simulink model "Pid"  (R2018a)
settings: Solver=VariableStepAuto  StartTime=0.0  StopTime=inf  RelTol=1e-3
undefined symbols (not defined in the file or in its folder): f
libraries: simulink x26, instrumentlib x3, aerolibanimutils x1
settings Model: Creator=user  LastModifiedBy=user

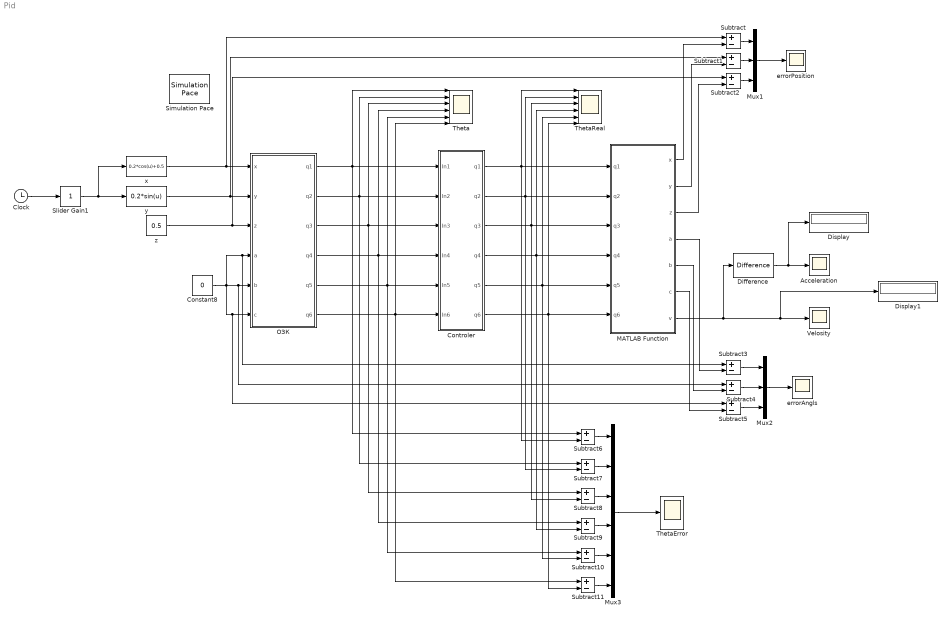
== system Pid ==
  Acceleration : Scope
  Clock : Clock
  Constant8 : Constant  Value=0
  Controler : Subsystem
  Difference : simulink/Discrete/Difference  ICPrevInput=0.0  OutMin=[]  OutMax=[]  OutDataType=fixdt(1, 16)  OutScaling=2^-10  DoSatur=off
  Display : Display
  Display1 : Display
  MATLAB Function : MATLAB Function  TreatAsAtomicUnit=on
  Mux1 : Mux  Inputs=3
  Mux2 : Mux  Inputs=3
  Mux3 : Mux  Inputs=6
  Simulation Pace : aerolibanimutils/Simulation Pace  SimulationPace=1  SleepMode=MATLAB Thread  OutputPaceError=off  SampleTime=1/200
  Slider Gain1 : simulink/Math Operations/Slider Gain  gain=1  low=0  high=10
  Subtract{,1..11} (12 alike) : Sum  Inputs=+-
  Theta : Scope  NumInputPorts=6
  ThetaError : Scope
  ThetaReal : Scope  NumInputPorts=6
  Velosity : Scope
  errorAngls : Scope
  errorPosition : Scope
  x : Fcn  Expr=0.2*cos(u)+0.5
  y : Fcn  Expr=0.2*sin(u)
  z : Constant  Value=0.5
  ОЗК : MATLAB Function  TreatAsAtomicUnit=on
  wires:
  Constant8/1 -> Subtract3/1, ОЗК/4(a), Subtract5/1, ОЗК/6(c), Subtract4/1, ОЗК/5(b)
  MATLAB Function/1(x) -> Subtract/2
  MATLAB Function/2(y) -> Subtract1/2
  MATLAB Function/3(z) -> Subtract2/2
  MATLAB Function/4(a) -> Subtract3/2
  MATLAB Function/5(b) -> Subtract4/2
  MATLAB Function/6(c) -> Subtract5/2
  ОЗК/1(q1) -> Subtract6/1, Controler/1(In1), Theta/1
  ОЗК/3(q3) -> Subtract8/1, Theta/3, Controler/3(In3)
  ОЗК/4(q4) -> Subtract9/1, Controler/4(In4), Theta/4
  ОЗК/2(q2) -> Subtract7/1, Controler/2(In2), Theta/2
  ОЗК/5(q5) -> Subtract10/1, Theta/5, Controler/5(In5)
  ОЗК/6(q6) -> Subtract11/1, Controler/6(In6), Theta/6
  z/1 -> Subtract2/1, ОЗК/3(z)
  y/1 -> Subtract1/1, ОЗК/2(y)
  x/1 -> Subtract/1, ОЗК/1(x)
  Controler/1("q1 ") -> Subtract6/2, ThetaReal/1, MATLAB Function/1(q1)
  Controler/2(q2) -> Subtract7/2, ThetaReal/2, MATLAB Function/2(q2)
  Controler/3(q3) -> Subtract8/2, ThetaReal/3, MATLAB Function/3(q3)
  Controler/4(q4) -> Subtract9/2, ThetaReal/4, MATLAB Function/4(q4)
  Controler/5(q5) -> Subtract10/2, ThetaReal/5, MATLAB Function/5(q5)
  Controler/6(q6) -> Subtract11/2, ThetaReal/6, MATLAB Function/6(q6)
  MATLAB Function/7(v) -> Difference/1, Display1/1, Velosity/1
  Difference/1 -> Display/1, Acceleration/1
  Subtract/1 -> Mux1/1
  Subtract1/1 -> Mux1/2
  Subtract2/1 -> Mux1/3
  Mux1/1 -> errorPosition/1
  Subtract4/1 -> Mux2/2
  Subtract3/1 -> Mux2/1
  Subtract5/1 -> Mux2/3
  Mux2/1 -> errorAngls/1
  Subtract6/1 -> Mux3/1
  Subtract7/1 -> Mux3/2
  Subtract8/1 -> Mux3/3
  Subtract9/1 -> Mux3/4
  Subtract10/1 -> Mux3/5
  Subtract11/1 -> Mux3/6
  Mux3/1 -> ThetaError/1
  Clock/1 -> Slider Gain1/1
  Slider Gain1/1 -> x/1, y/1

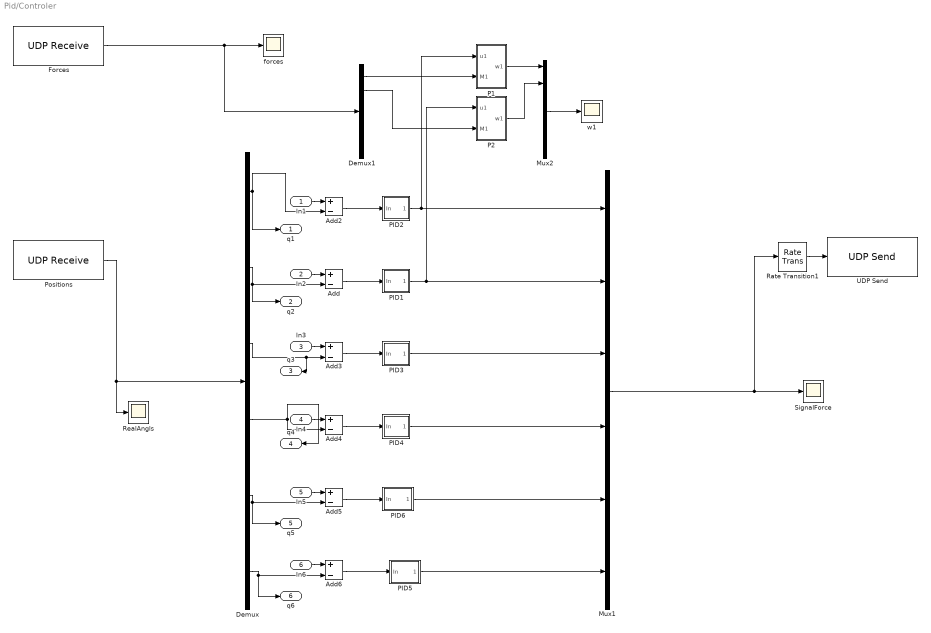
== system Pid/Controler ==
  In1 : Inport
  In2 : Inport  Port=2
  In3 : Inport  Port=3
  In4 : Inport  Port=4
  In5 : Inport  Port=5
  In6 : Inport  Port=6
  Add{,2..6} (6 alike) : Sum  Inputs=+-
  Demux : Demux  Outputs=6
  Demux1 : Demux  Outputs=6
  Forces : instrumentlib/UDP Receive  Host=localhost  Port=20005  LocalPort=20005  EnablePortSharing=off  GetLatestData=off  DataSize=6  DataType=double  ASCIIFormatting=%f,  Terminator=LF  ByteOrder=LittleEndian  EnableBlockingMode=on  Timeout=10  SampleTime=0.01  LocalAddress=localhost
      settings: SourceProductName=Instrument Control Toolbox
  Mux1 : Mux  Inputs=6
  Mux2 : Mux  Inputs=6
  P1 : Subsystem
  P2 : Subsystem
  PID1 : Subsystem
  PID2 : Subsystem
  PID3 : Subsystem
  PID4 : Subsystem
  PID5 : Subsystem
  PID6 : Subsystem
  Positions : instrumentlib/UDP Receive  Host=localhost  Port=20001  LocalPort=20001  EnablePortSharing=off  GetLatestData=off  DataSize=6  DataType=double  ASCIIFormatting=%f,  Terminator=LF  ByteOrder=LittleEndian  EnableBlockingMode=on  Timeout=10  SampleTime=0.01  LocalAddress=localhost
      settings: SourceProductName=Instrument Control Toolbox
  Rate Transition1 : RateTransition  OutPortSampleTime=0.01
  RealAngls : Scope
  SignalForce : Scope
  UDP Send : instrumentlib/UDP Send  Host=localhost  Port=20000  LocalPort=-1  EnablePortSharing=off  ByteOrder=LittleEndian  OutputDatagramPacketSize=512  EnableBlockingMode=on  LocalAddress=0.0.0.0
      settings: SourceProductName=Instrument Control Toolbox
  forces : Scope
  w1 : Scope
  "q1 " : Outport
  q2 : Outport  Port=2
  q3 : Outport  Port=3
  q4 : Outport  Port=4
  q5 : Outport  Port=5
  q6 : Outport  Port=6
  wires:
  Mux1/1 -> Rate Transition1/1, SignalForce/1
  In4/1 -> Add4/1
  In5/1 -> Add5/1
  Rate Transition1/1 -> UDP Send/1
  In3/1 -> Add3/1
  In1/1 -> Add2/1
  In6/1 -> Add6/1
  In2/1 -> Add/1
  PID2/1("out1 ") -> P1/1(u1), Mux1/1
  PID1/1("out1 ") -> P2/1(u1), Mux1/2
  PID3/1("out1 ") -> Mux1/3
  PID4/1("out1 ") -> Mux1/4
  PID6/1("out1 ") -> Mux1/5
  PID5/1("out1 ") -> Mux1/6
  Add/1 -> PID1/1(In)
  Add2/1 -> PID2/1(In)
  Add3/1 -> PID3/1(In)
  Add4/1 -> PID4/1(In)
  Add5/1 -> PID6/1(In)
  Add6/1 -> PID5/1(In)
  P1/1(w1) -> Mux2/1
  Mux2/1 -> w1/1
  Demux1/2 -> P2/2(M1)
  P2/1(w1) -> Mux2/2
  Positions/1 -> Demux/1, RealAngls/1
  Forces/1 -> Demux1/1, forces/1
  Demux/1 -> Add2/2, "q1 "/1
  Demux/2 -> Add/2, q2/1
  Demux/3 -> Add3/2, q3/1
  Demux/4 -> q4/1, Add4/2
  Demux/5 -> Add5/2, q5/1
  Demux/6 -> Add6/2, q6/1
  Demux1/1 -> P1/2(M1)

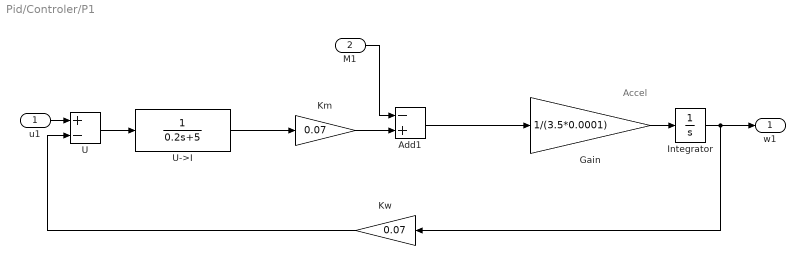
== system Pid/Controler/P1 ==
  note: Accel
  u1 : Inport
  M1 : Inport  Port=2
  Add1 : Sum  Inputs=-+
  Gain : Gain  Gain=1/(3.5*0.0001)
  Integrator : Integrator
  Km : Gain  Gain=0.07
  Kw : Gain  Gain=0.07
  U : Sum  Inputs=+-
  U->I : TransferFcn  Denominator=[0.2 5]
  w1 : Outport
  wires:
  U->I/1 -> Km/1
  Km/1 -> Add1/2
  u1/1 -> U/1
  Integrator/1 -> w1/1, Kw/1
  Kw/1 -> U/2
  U/1 -> U->I/1
  Gain/1 -> Integrator/1
  Add1/1 -> Gain/1
  M1/1 -> Add1/1

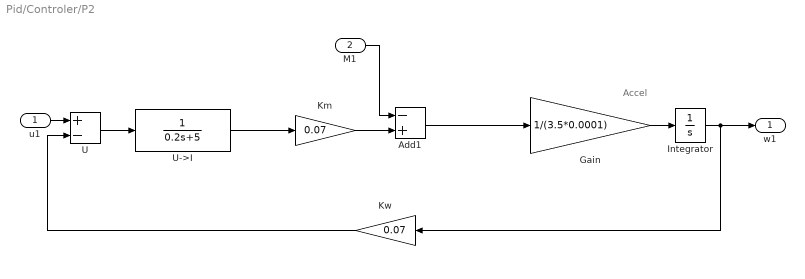
== system Pid/Controler/P2 ==
  note: Accel
  u1 : Inport
  M1 : Inport  Port=2
  Add1 : Sum  Inputs=-+
  Gain : Gain  Gain=1/(3.5*0.0001)
  Integrator : Integrator
  Km : Gain  Gain=0.07
  Kw : Gain  Gain=0.07
  U : Sum  Inputs=+-
  U->I : TransferFcn  Denominator=[0.2 5]
  w1 : Outport
  wires:
  M1/1 -> Add1/1
  Add1/1 -> Gain/1
  Gain/1 -> Integrator/1
  U/1 -> U->I/1
  Kw/1 -> U/2
  Integrator/1 -> Kw/1, w1/1
  u1/1 -> U/1
  Km/1 -> Add1/2
  U->I/1 -> Km/1

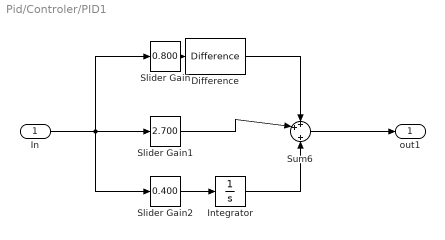
== system Pid/Controler/PID1 ==
  In : Inport
  Difference : simulink/Discrete/Difference  ICPrevInput=0.0  OutMin=[]  OutMax=[]  OutDataType=fixdt(1, 16)  OutScaling=2^-10  DoSatur=off
  Integrator : Integrator
  Slider Gain : simulink/Math Operations/Slider Gain  gain=0.800  low=0  high=10
  Slider Gain1 : simulink/Math Operations/Slider Gain  gain=2.700  low=0  high=10
  Slider Gain2 : simulink/Math Operations/Slider Gain  gain=0.400  low=0  high=10
  Sum6 : Sum  Inputs=++|+
  "out1 " : Outport
  wires:
  Slider Gain1/1 -> Sum6/2
  Integrator/1 -> Sum6/3
  Slider Gain2/1 -> Integrator/1
  Slider Gain/1 -> Difference/1
  Sum6/1 -> "out1 "/1
  Difference/1 -> Sum6/1
  In/1 -> Slider Gain1/1, Slider Gain/1, Slider Gain2/1

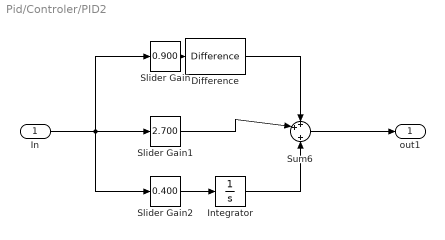
== system Pid/Controler/PID2 ==
  In : Inport
  Difference : simulink/Discrete/Difference  ICPrevInput=0.0  OutMin=[]  OutMax=[]  OutDataType=fixdt(1, 16)  OutScaling=2^-10  DoSatur=off
  Integrator : Integrator
  Slider Gain : simulink/Math Operations/Slider Gain  gain=0.900  low=0  high=10
  Slider Gain1 : simulink/Math Operations/Slider Gain  gain=2.700  low=0  high=10
  Slider Gain2 : simulink/Math Operations/Slider Gain  gain=0.400  low=0  high=10
  Sum6 : Sum  Inputs=++|+
  "out1 " : Outport
  wires:
  In/1 -> Slider Gain2/1, Slider Gain/1, Slider Gain1/1
  Difference/1 -> Sum6/1
  Sum6/1 -> "out1 "/1
  Slider Gain/1 -> Difference/1
  Slider Gain2/1 -> Integrator/1
  Integrator/1 -> Sum6/3
  Slider Gain1/1 -> Sum6/2

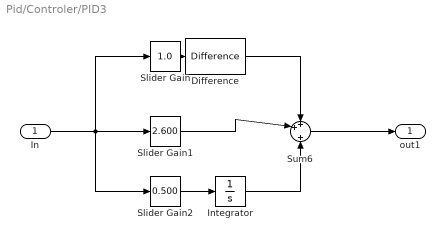
== system Pid/Controler/PID3 ==
  In : Inport
  Difference : simulink/Discrete/Difference  ICPrevInput=0.0  OutMin=[]  OutMax=[]  OutDataType=fixdt(1, 16)  OutScaling=2^-10  DoSatur=off
  Integrator : Integrator
  Slider Gain : simulink/Math Operations/Slider Gain  gain=1.0  low=0  high=10
  Slider Gain1 : simulink/Math Operations/Slider Gain  gain=2.600  low=0  high=10
  Slider Gain2 : simulink/Math Operations/Slider Gain  gain=0.500  low=0  high=10
  Sum6 : Sum  Inputs=++|+
  "out1 " : Outport
  wires:
  In/1 -> Slider Gain2/1, Slider Gain/1, Slider Gain1/1
  Difference/1 -> Sum6/1
  Sum6/1 -> "out1 "/1
  Slider Gain/1 -> Difference/1
  Slider Gain2/1 -> Integrator/1
  Integrator/1 -> Sum6/3
  Slider Gain1/1 -> Sum6/2

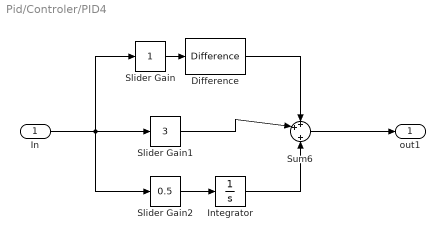
== system Pid/Controler/PID4 ==
  In : Inport
  Difference : simulink/Discrete/Difference  ICPrevInput=0.0  OutMin=[]  OutMax=[]  OutDataType=fixdt(1, 16)  OutScaling=2^-10  DoSatur=off
  Integrator : Integrator
  Slider Gain : simulink/Math Operations/Slider Gain  gain=1  low=0  high=10
  Slider Gain1 : simulink/Math Operations/Slider Gain  gain=3  low=0  high=10
  Slider Gain2 : simulink/Math Operations/Slider Gain  gain=0.5  low=0  high=10
  Sum6 : Sum  Inputs=++|+
  "out1 " : Outport
  wires:
  Slider Gain1/1 -> Sum6/2
  Integrator/1 -> Sum6/3
  Slider Gain2/1 -> Integrator/1
  Slider Gain/1 -> Difference/1
  Sum6/1 -> "out1 "/1
  Difference/1 -> Sum6/1
  In/1 -> Slider Gain1/1, Slider Gain/1, Slider Gain2/1

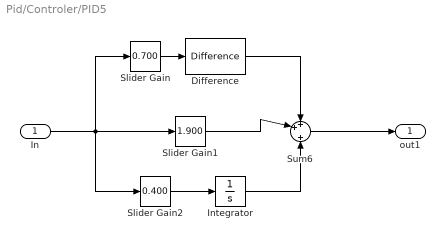
== system Pid/Controler/PID5 ==
  In : Inport
  Difference : simulink/Discrete/Difference  ICPrevInput=0.0  OutMin=[]  OutMax=[]  OutDataType=fixdt(1, 16)  OutScaling=2^-10  DoSatur=off
  Integrator : Integrator
  Slider Gain : simulink/Math Operations/Slider Gain  gain=0.700  low=0  high=10
  Slider Gain1 : simulink/Math Operations/Slider Gain  gain=1.900  low=0  high=10
  Slider Gain2 : simulink/Math Operations/Slider Gain  gain=0.400  low=0  high=10
  Sum6 : Sum  Inputs=++|+
  "out1 " : Outport
  wires:
  Slider Gain1/1 -> Sum6/2
  Integrator/1 -> Sum6/3
  Slider Gain2/1 -> Integrator/1
  Slider Gain/1 -> Difference/1
  Sum6/1 -> "out1 "/1
  Difference/1 -> Sum6/1
  In/1 -> Slider Gain/1, Slider Gain1/1, Slider Gain2/1

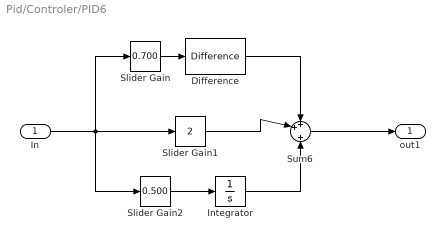
== system Pid/Controler/PID6 ==
  In : Inport
  Difference : simulink/Discrete/Difference  ICPrevInput=0.0  OutMin=[]  OutMax=[]  OutDataType=fixdt(1, 16)  OutScaling=2^-10  DoSatur=off
  Integrator : Integrator
  Slider Gain : simulink/Math Operations/Slider Gain  gain=0.700  low=0  high=10
  Slider Gain1 : simulink/Math Operations/Slider Gain  gain=2  low=0  high=10
  Slider Gain2 : simulink/Math Operations/Slider Gain  gain=0.500  low=0  high=10
  Sum6 : Sum  Inputs=++|+
  "out1 " : Outport
  wires:
  In/1 -> Slider Gain2/1, Slider Gain1/1, Slider Gain/1
  Difference/1 -> Sum6/1
  Sum6/1 -> "out1 "/1
  Slider Gain/1 -> Difference/1
  Slider Gain2/1 -> Integrator/1
  Integrator/1 -> Sum6/3
  Slider Gain1/1 -> Sum6/2

== matlab function Pid/ОЗК ==
  data: x input; q1 output; y input; z input; q2 output; q3 output; a input; b input; c input; q4 output; q5 output; q6 output
function [q1,q2,q3,q4,q5,q6] = InverseKinematics(x,y,z,a,b,c)
%This function is used for inverse kinematics calculations.

%link lenghts in mm


% d1=0.4865;
% d2=0.150;
% d3=0.475;
% d4=0.600;
% d6=0.065;
d1 = 0.352;
d2 = 0.070;
d3 = 0.360;
d4 = 0.380;
d6=0.065;

alpha = [ 0,-pi/2, 0, -pi/2, pi/2, -pi/2];
% a = [d2 d3 0 0 0 0];
% d = [d1 0 0 d4 0 d6];

%%%%%%%%%%%%%%%%%Inverse kinematics%%%%%%%%%%%%%%%%%

R06= [cos(a)*cos(b), cos(a)*sin(c)*sin(b)-sin(a)*cos(c), cos(a)*sin(b)*cos(c)+sin(a)*sin(c);
      sin(a)*cos(b), sin(a)*sin(b)*sin(c)+cos(a)*cos(c), sin(a)*sin(b)*cos(c)-cos(a)*sin(c);
      - sin(b),      cos(b)*sin(c),                      cos(b)*cos(c)];


p06=[x y z];
p04=p06-transpose(d6*R06*[0;0;1]);

xc=p04(1);
yc=p04(2);
zc=p04(3);



%Inverse kinematic equations for position
theta1 = atan2(yc,xc);

r = (xc^2 + yc^2)^(1/2);
COS = ((r - d2)^2 + (zc - d1)^2 - d3^2 - d4^2)/(2*d3*d4);

theta3_dash = atan2((-(1 - COS^2)^(1/2)), COS);
theta3 = theta3_dash;
theta33 = abs(theta3_dash) - (90*pi/180);

theta2_dash = (atan2( zc-d1, r-d2) - atan2(d4*sind(theta3_dash*180/pi),d3+d4*cosd(theta3_dash*180/pi))) ;
theta2 = theta2_dash;
theta22 = (90*pi/180) - theta2_dash;

theta5 = atan2(sqrt(1-(sin(theta1)*R06(1,3)- cos(theta1)*R06(2,3))^2),sin(theta1)*R06(1,3) - cos(theta1)*R06(2,3)) -pi;
% theta4 = atan2(-cos(theta1)*sin(theta22+theta33)*R06(1,3)-sin(theta1)*sin(theta22+theta33)*R06(2,3)+cos(theta22+theta33)*R06(3,3),cos(theta1)*cos(theta22+theta33)*R06(1,3)+sin(theta1)*cos(theta22+theta33)*R06(2,3)+sin(theta22+theta33)*R06(3,3));
theta4 = atan2(-cos(theta1)*sin(theta2+theta3)*R06(1,3)-sin(theta1)*sin(theta2+theta3)*R06(2,3)+cos(theta2+theta3)*R06(3,3),cos(theta1)*cos(theta2+theta3)*R06(1,3)+sin(theta1)*cos(theta2+theta3)*R06(2,3)+sin(theta2+theta3)*R06(3,3));
theta6= atan2(sin(theta1)*R06(1,2)-cos(theta1)*R06(2,2),-sin(theta1)*R06(1,1)+cos(theta1)*R06(2,1));

%%Theta 4 изменен

% R30 = [cos(theta1).*cos(theta2+theta3), -cos(theta1).*sin(theta2+theta3), sin(theta1);
%  sin(theta1).*cos(theta2+theta3), -sin(theta1).*sin(theta2+theta3), cos(theta1);
%  -sin(theta2+theta3), -cos(theta2+theta3), 0 ] ;

R03=[ cos(theta1)*cos(theta2)*cos(theta3) - cos(theta1)*sin(theta2)*sin(theta3), - cos(theta1)*cos(theta2)*sin(theta3) - cos(theta1)*cos(theta3)*sin(theta2), -sin(theta1);
 cos(theta2)*cos(theta3)*sin(theta1) - sin(theta1)*sin(theta2)*sin(theta3), - cos(theta2)*sin(theta1)*sin(theta3) - cos(theta3)*sin(theta1)*sin(theta2),  cos(theta1);
     - cos(theta2)*sin(theta3) - cos(theta3)*sin(theta2),         sin(theta2)*sin(theta3) - cos(theta2)*cos(theta3),   0];

 RT03= transpose (R03);
 
R36 = RT03 * R06 ;
g11 = R36 (1,1);
g12 = R36 (1,2);
g23 = R36 (2,3);
g13 = R36 (1,3);
g22 = R36 (2,2);
g33 = R36 (3,3);
g21 = R36 (2,1);

        Q5 = atan2 ( sqrt(1-g23^2), g23)-pi/2;
if(Q5 == 0)
    Q4= 0;
    Q6 = atan2 (-g12, g11);
Q5=0.00000000001;
elseif (Q5 == pi)

     Q4= 0;
     Q5= 0;
     Q6 = atan2 (g12,-g11);
else
    Q4 = atan2 (g33/ sin (Q5), - g13/ sin (Q5));
    Q6 = atan2 (g22/ -sin (Q5), g21/ sin (Q5));
end

q1=theta1;
q2=theta2;
q3=theta3;
q4=Q4;
q5=Q5;
q6=Q6;


end

== matlab function Pid/MATLAB Function ==
  data: q1 input; x output; y output; z output; a output; b output; c output; q2 input; q3 input; q4 input; q5 input; q6 input; v output
function [x,y,z,a,b,c,v] = ForvardKinematics(q1,q2,q3,q4,q5,q6)

%   i       Link twist     Link Length     Link Offset    Joint Angle    
%--------------------------------------------------------------------------
%   1        -90              d2             d1                 theta1*     
%   2         0               d3              0               theta2 - 90*  
%   3        -90               0              0                 theta3*     
%   4         90               0             d4                 theta4*     
%   5        -90               0              0                 theta5*     
%   6         0                0             d5                 theta6*     

Jacobian = [];
J = zeros(6,6);
V=zeros(3,6);
w=zeros(3,6);

d1 = 0.352;
d2 = 0.070;
d3 = 0.360;
d4 = 0.380;
d6=0.065;

q1=q1*180/pi;
q2=q2*180/pi;
q3=q3*180/pi;
q4=q4*180/pi;
q5=q5*180/pi;
q6=q6*180/pi;

T01 = make_tfMatrix(d2, -90, q1 ,d1);  
T12 = make_tfMatrix(d3,  0, q2 ,   0);
T23 = make_tfMatrix(0, -90,     q3-90    ,0);
T34 = make_tfMatrix(0,  90,      q4    , d4); 
T45 = make_tfMatrix(0, -90,      q5    , 0);
T56 = make_tfMatrix(0,   0,      q6    , d6);

% T06=T01*T12*T23*T34*T45*T56;
T02=T01*T12;
T03=T02*T23;
T04=T03*T34;
T05=T04*T45;
T06=T05*T56;

p00=[0;0;0];
p01=T01(1:3,4);
p02=T02(1:3,4);
p03=T03(1:3,4);
p04=T04(1:3,4);
p05=T05(1:3,4);
p06=T06(1:3,4);

z0 = [0;0;1];
z1 = T01(1:3,1:3)*[0;0;1];
z2 = T02(1:3,1:3)*[0;0;1];
z3 = T03(1:3,1:3)*[0;0;1];
z4 = T04(1:3,1:3)*[0;0;1];
z5 = T05(1:3,1:3)*[0;0;1];
z6 = T06(1:3,1:3)*[0;0;1];


J(:,1) = [cross(z0,(p06 - p00));z0];
J(:,2) = [cross(z1,(p06 - p01));z2];
J(:,3) = [cross(z2,(p06 - p02));z3];
J(:,4) = [cross(z3,(p06 - p03));z4];
J(:,5) = [cross(z4,(p06 - p04));z5];
J(:,6) = [cross(z5,(p06 - p05));z6];

Jacobian = cat(3, Jacobian, J);

for i = 1 : 6
    V(1, :) = Jacobian(1, i, :);
    V(2, :) = Jacobian(2, i, :);
    V(3, :) = Jacobian(3, i, :);
    w(1, :) = Jacobian(4, i, :);
    w(2, :) = Jacobian(5, i, :);
    w(3, :) = Jacobian(6, i, :); 
end

v06=transpose(V(1:3,6));

v=sqrt(v06(1)^2+v06(2)^2+v06(3)^2);

x=p06(1);
y=p06(2);
z=p06(3);


R06=T06(1:3,1:3);


if R06(3,3)==1
    a=0;
    c=0;
    b=atan2(R06(2,1),R06(1,1));
elseif R06(3,3)==-1
     a=0;
     c=0;
     b=atan2(-R06(1,2),-R06(1,1));
else
    a=atan2(R06(2,3),R06(1,3));
    b=atan2(R06(3,2),-R06(3,1));
    c=atan2(sqrt(abs(1-R06(3,3)^2)),R06(3,3));
end

function [ transformation_matrix ] = make_tfMatrix( a, alpha, th, d )


transformation_matrix = [cosd(th),   -sind(th)*cosd(alpha),      sind(th)*sind(alpha),      a*cosd(th);
                         sind(th),    cosd(th)*cosd(alpha),     -cosd(th)*sind(alpha),      a*sind(th);
                              0  ,          sind(alpha)   ,          cosd(alpha)     ,           d    ;
                              0  ,             0          ,               0          ,            1   ];

end
    
end
